simulink model "H2_LQG_quarter_Car"  (R2025b)
settings: Solver=VariableStepAuto  StartTime=0.0  StopTime=30  RelTol=1e-3
values from neighbouring files (symbols this model uses):
  omega_n1 = 80    [A_quarter_car_parameters.m]    (also in A_uncertain_Plant.m = parameters.omega_n1; Incert_plant.m; LQG.m; LQG_pt2.m)
  tau_1 = 0.005    [A_quarter_car_parameters.m]    (also in LQG.m; LQG_pt2.m; LQG_pt2.mat; Lin_model.m)
  tau_2 = 0.010    (= 0.01)    [A_quarter_car_parameters.m]    (also in LQG.m; LQG_pt2.m; LQG_pt2.mat; Lin_model.m)
  tau_a = 0.025    [A_quarter_car_parameters.m]    (also in A_uncertain_Plant.m = parameters.tau_a; Incert_plant.m; LQG.m; LQG_pt2.m)
  x0_delta_s = 0    [A_quarter_car_parameters.m]    (also in quarter_car_parameters.m)
  x0_delta_t = 0    [A_quarter_car_parameters.m]    (also in quarter_car_parameters.m)
  x0_zs_dot = 0    [A_quarter_car_parameters.m]    (also in quarter_car_parameters.m)
  x0_zu_dot = 0    [A_quarter_car_parameters.m]    (also in quarter_car_parameters.m)
  zeta_1 = 0.7    [A_quarter_car_parameters.m]    (also in A_uncertain_Plant.m = parameters.zeta_1; Incert_plant.m; LQG.m; LQG_pt2.m)
libraries: simulink x4, cstblocks x3
settings Model: Creator=ettor  LastModifiedBy=ettor

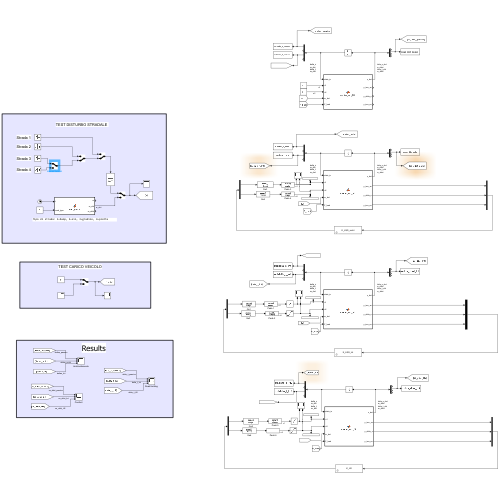
[thumbnail: Simulink's stored preview of the top-level diagram]
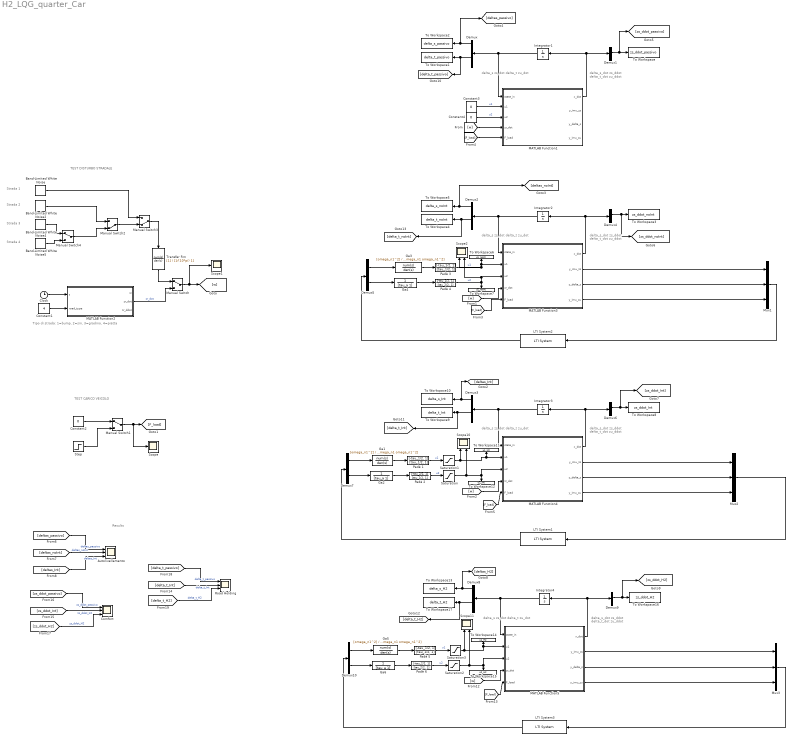
== system H2_LQG_quarter_Car ==
  note: Results
  note: Tipo di strada: 1=bump, 2=sin, 3=gradino, 4=piatta
  note: TEST CARICO VEICOLO
  note: delta_s
      | zs_dot
      | delta_t
      | zu_dot
  note: delta_s_dot
      | zs_ddot
      | delta_t_dot
      | zu_ddot
  note: delta_s_dot
      | zs_ddot
      | delta_t_dot
      | zu_ddot
  note: TEST DISTURBO STRADALE
  note: delta_s_dot
      | zs_ddot
      | delta_t_dot
      | zu_ddot
  note: delta_s
      | zs_dot
      | delta_t
      | zu_dot
  note: delta_s
      | zs_dot
      | delta_t
      | zu_dot
  note: delta_s_dot
      | zs_ddot
      | delta_t_dot
      | zu_ddot
  note: delta_s
      | zs_dot
      | delta_t
      | zu_dot
  note: Strada 2
  note: Strada 3
  note: Strada 4
  note: Strada 1
  Autolivellamento : Scope  NumInputPorts=3
      settings: ActiveDisplayYMinimum=-0.18076927505597792  ActiveDisplayYMaximum=0.021014396276541246  YLabel=[m]  DataLoggingVariableName=ScopeData2
  Band-Limited White Noise : simulink/Sources/Band-Limited White Noise  Cov=[5e-3*0.01]  Ts=0.01  seed=[23341]
  Band-Limited White Noise2 : simulink/Sources/Band-Limited White Noise  Cov=[6e-2*0.01]  Ts=0.01  seed=[23341]
  Band-Limited White Noise4 : simulink/Sources/Band-Limited White Noise  Cov=[0.15*0.01]  Ts=0.01  seed=[23341]
  Band-Limited White Noise5 : simulink/Sources/Band-Limited White Noise  Cov=[0.30*0.01]  Ts=0.01  seed=[23341]
  Clock : Clock
  "Comfort " : Scope  NumInputPorts=3
      settings: ActiveDisplayYMinimum=-3.7790657356038841  ActiveDisplayYMaximum=3.5650054973377014  YLabel=[m/s^2]  DataLoggingVariableName=ScopeData8
  Constant1 : Constant  Value=4
  Constant2 : Constant  Value=0
  Constant3 : Constant  Value=0
  Constant4 : Constant  Value=0
  Demux{,1..4,6,8..9} (8 alike) : Demux
  Demux10 : Demux  Outputs=2
  Demux5 : Demux  Outputs=2
  Demux7 : Demux  Outputs=2
  Ga1 : TransferFcn  Numerator=[omega_n1^2]  Denominator=[1 2*zeta_1*omega_n1 omega_n1^2]
  Ga2 : TransferFcn  Denominator=[tau_a 1]
  Ga3 : TransferFcn  Numerator=[omega_n1^2]  Denominator=[1 2*zeta_1*omega_n1 omega_n1^2]
  Ga4 : TransferFcn  Denominator=[tau_a 1]
  Ga5 : TransferFcn  Numerator=[omega_n1^2]  Denominator=[1 2*zeta_1*omega_n1 omega_n1^2]
  Ga6 : TransferFcn  Denominator=[tau_a 1]
  Integrator{1..4} (4 alike) : Integrator  InitialCondition=[x0_delta_s; x0_zs_dot; x0_delta_t; x0_zu_dot]
  LTI System1 : cstblocks/LTI System  sys=K_LQG_Int  IC=[]  PadeOrder=0
  LTI System2 : cstblocks/LTI System  sys=K_LQG_noInt  IC=[]  PadeOrder=0
  LTI System3 : cstblocks/LTI System  sys=K_H2  IC=[]  PadeOrder=0
  MATLAB Function1 : MATLAB Function  TreatAsAtomicUnit=on
  MATLAB Function2 : MATLAB Function  TreatAsAtomicUnit=on
  MATLAB Function3 : MATLAB Function  TreatAsAtomicUnit=on
  MATLAB Function4 : MATLAB Function  TreatAsAtomicUnit=on
  MATLAB Function5 : MATLAB Function  TreatAsAtomicUnit=on
  Manual Switch : ManualSwitch
  Manual Switch1 : ManualSwitch
  Manual Switch2 : ManualSwitch  CurrentSetting=0
  Manual Switch3 : ManualSwitch  CurrentSetting=0
  Manual Switch4 : ManualSwitch
  Mux1 : Mux  Inputs=3
  Mux2 : Mux  Inputs=3
  Mux3 : Mux  Inputs=3
  Padè 1 : TransferFcn  Numerator=[-tau_1/2, 1]  Denominator=[tau_1/2, 1]
  Padè 2 : TransferFcn  Numerator=[-tau_2/2, 1]  Denominator=[tau_2/2, 1]
  Padè 3 : TransferFcn  Numerator=[-tau_1/2, 1]  Denominator=[tau_1/2, 1]
  Padè 4 : TransferFcn  Numerator=[-tau_2/2, 1]  Denominator=[tau_2/2, 1]
  Padè 5 : TransferFcn  Numerator=[-tau_1/2, 1]  Denominator=[tau_1/2, 1]
  Padè 6 : TransferFcn  Numerator=[-tau_2/2, 1]  Denominator=[tau_2/2, 1]
  "Road Holding " : Scope  NumInputPorts=3
      settings: ActiveDisplayYMinimum=-0.017632393466422407  ActiveDisplayYMaximum=0.022207758401506367  YLabel=[m]  DataLoggingVariableName=ScopeData11
  Saturation : Saturate  UpperLimit=+3000  LowerLimit=-3000
  Saturation1 : Saturate  UpperLimit=+3000  LowerLimit=-3000
  Saturation2 : Saturate  UpperLimit=+10000  LowerLimit=-10000
  Saturation3 : Saturate  UpperLimit=+5000  LowerLimit=-5000
  Scope : Scope
      settings: ActiveDisplayYMinimum=-1  ActiveDisplayYMaximum=1
  Scope1 : Scope
      settings: ActiveDisplayYMinimum=-1  ActiveDisplayYMaximum=1
  Scope10 : Scope  NumInputPorts=2
      settings: ActiveDisplayYMinimum=-1  ActiveDisplayYMaximum=1  DataLoggingVariableName=ScopeData9
  Scope11 : Scope  NumInputPorts=2
      settings: ActiveDisplayYMinimum=-103.06262892158483  ActiveDisplayYMaximum=567.88180424316226  DataLoggingVariableName=ScopeData10
  Scope2 : Scope  NumInputPorts=2
      settings: ActiveDisplayYMinimum=-1  ActiveDisplayYMaximum=1  DataLoggingVariableName=ScopeData3
  Step : Step  After=1000  SampleTime=0
  To Workspace : ToWorkspace  VariableName=zs_ddot_passivo  SaveFormat=Timeseries  SampleTime=-1
  To Workspace1 : ToWorkspace  VariableName=delta_t_passivo  SaveFormat=Timeseries  SampleTime=-1
  To Workspace10 : ToWorkspace  VariableName=delta_s_Int  SaveFormat=Timeseries  SampleTime=-1
  To Workspace11 : ToWorkspace  VariableName=u1_Int  SaveFormat=Timeseries  SampleTime=-1
  To Workspace12 : ToWorkspace  VariableName=u2_Int  SaveFormat=Timeseries  SampleTime=-1
  To Workspace13 : ToWorkspace  VariableName=delta_s_H2  SaveFormat=Timeseries  SampleTime=-1
  To Workspace14 : ToWorkspace  VariableName=u1_H2  SaveFormat=Timeseries  SampleTime=-1
  To Workspace15 : ToWorkspace  VariableName=u2_H2  SaveFormat=Timeseries  SampleTime=-1
  To Workspace16 : ToWorkspace  VariableName=zs_ddot_H2  SaveFormat=Timeseries  SampleTime=-1
  To Workspace17 : ToWorkspace  VariableName=delta_t_H2  SaveFormat=Timeseries  SampleTime=-1
  To Workspace2 : ToWorkspace  VariableName=delta_s_passivo  SaveFormat=Timeseries  SampleTime=-1
  To Workspace3 : ToWorkspace  VariableName=zs_ddot_noInt  SaveFormat=Timeseries  SampleTime=-1
  To Workspace4 : ToWorkspace  VariableName=delta_t_noInt  SaveFormat=Timeseries  SampleTime=-1
  To Workspace5 : ToWorkspace  VariableName=delta_s_noInt  SaveFormat=Timeseries  SampleTime=-1
  To Workspace6 : ToWorkspace  VariableName=u1_noInt  SaveFormat=Timeseries  SampleTime=-1
  To Workspace7 : ToWorkspace  VariableName=u2_noInt  SaveFormat=Timeseries  SampleTime=-1
  To Workspace8 : ToWorkspace  VariableName=zs_ddot_Int  SaveFormat=Timeseries  SampleTime=-1
  To Workspace9 : ToWorkspace  VariableName=delta_t_Int  SaveFormat=Timeseries  SampleTime=-1
  Transfer Fcn : TransferFcn  Denominator=[1/(10*pi) 1]
  wires:
  Manual Switch1/1 -> Scope/1, [F_load]
  Ga3/1 -> Padè 3/1
  Step/1 -> Manual Switch1/2
  Demux5/2 -> Ga4/1
  Saturation1/1 -> To Workspace11/1, MATLAB Function4/2(u1), Scope10/1
  Padè 1/1 -> Saturation1/1  "u1"
  Demux3/1 -> [deltas_Int], To Workspace10/1
  Demux3/3 -> [delta_t_Int], To Workspace9/1
  Demux2/1 -> [deltas_noInt], To Workspace5/1
  Demux7/2 -> Ga2/1
  Demux4/2 -> [zs_ddot_noInt], To Workspace3/1
  Constant2/1 -> Manual Switch1/1
  MATLAB Function2/2(zr_dot) -> Manual Switch/2  "zr_dot"
  [F_load] -> MATLAB Function4/5(F_load)
  Mux1/1 -> LTI System2/1
  MATLAB Function1/1(x_dot) -> Integrator1/1, Demux1/1
  Demux/1 -> [deltas_passivo], To Workspace2/1
  Integrator2/1 -> MATLAB Function3/1(state_in), Demux2/1
  Ga1/1 -> Padè 1/1
  Saturation/1 -> To Workspace12/1, MATLAB Function4/3(u2), Scope10/2
  [w] -> MATLAB Function3/4(zr_dot)
  Demux5/1 -> Ga3/1
  Demux/3 -> [delta_t_passivo], To Workspace1/1
  Integrator1/1 -> MATLAB Function1/1(state_in), Demux/1
  Demux6/2 -> [zs_ddot_Int], To Workspace8/1
  Constant1/1 -> MATLAB Function2/2(road_type)
  Constant4/1 -> MATLAB Function1/3(u2)  "u2"
  MATLAB Function3/1(x_dot) -> Demux4/1, Integrator2/1
  LTI System2/1 -> Demux5/1
  Padè 4/1 -> Scope2/2, MATLAB Function3/3(u2), To Workspace7/1  "u2"
  Padè 2/1 -> Saturation/1  "u2"
  [w] -> MATLAB Function4/4(zr_dot)
  Ga2/1 -> Padè 2/1
  Constant3/1 -> MATLAB Function1/2(u1)  "u1"
  [F_load] -> MATLAB Function3/5(F_load)
  [F_load] -> MATLAB Function1/5(F_load)
  Padè 3/1 -> Scope2/1, To Workspace6/1, MATLAB Function3/2(u1)  "u1"
  [w] -> MATLAB Function1/4(zr_dot)
  Mux2/1 -> LTI System1/1
  Demux2/3 -> [delta_t_noInt], To Workspace4/1
  Integrator3/1 -> MATLAB Function4/1(state_in), Demux3/1
  Demux7/1 -> Ga1/1
  Clock/1 -> MATLAB Function2/1(t)
  Demux1/2 -> [zs_ddot_passivo], To Workspace/1
  MATLAB Function4/1(x_dot) -> Demux6/1, Integrator3/1
  Ga4/1 -> Padè 4/1
  LTI System1/1 -> Demux7/1
  Manual Switch/1 -> Scope1/1, [w]
  [deltas_passivo] -> Autolivellamento/1  "deltas_passivo"
  [deltas_noInt] -> Autolivellamento/2  "deltas_noInt"
  [deltas_Int] -> Autolivellamento/3  "deltas_Int"
  Band-Limited White Noise/1 -> Manual Switch3/1
  Band-Limited White Noise2/1 -> Manual Switch2/1
  Manual Switch2/1 -> Manual Switch3/2
  Manual Switch3/1 -> Transfer Fcn/1
  Ga5/1 -> Padè 5/1
  [F_load] -> MATLAB Function5/5(F_load)
  Demux10/2 -> Ga6/1
  Demux8/3 -> [delta_t_H2], To Workspace17/1
  Saturation2/1 -> MATLAB Function5/3(u2), To Workspace15/1, Scope11/2
  Demux8/1 -> [deltas_H2], To Workspace13/1
  Padè 5/1 -> Saturation3/1  "u1"
  Saturation3/1 -> To Workspace14/1, MATLAB Function5/2(u1), Scope11/1
  Demux10/1 -> Ga5/1
  Integrator4/1 -> MATLAB Function5/1(state_in), Demux8/1
  Mux3/1 -> LTI System3/1
  Ga6/1 -> Padè 6/1
  Padè 6/1 -> Saturation2/1  "u2"
  Demux9/2 -> [zs_ddot_H2], To Workspace16/1
  LTI System3/1 -> Demux10/1
  MATLAB Function5/1(x_dot) -> Demux9/1, Integrator4/1
  [w] -> MATLAB Function5/4(zr_dot)
  [zs_ddot_passivo] -> "Comfort "/1  "zs_ddot_passivo"
  [zs_ddot_Int] -> "Comfort "/2  "zs_ddot_Int"
  [zs_ddot_H2] -> "Comfort "/3  "zs_ddot_H2"
  [delta_t_passivo] -> "Road Holding "/1  "delta_t_passivo"
  [delta_t_Int] -> "Road Holding "/2  "delta_t_Int"
  [delta_t_H2] -> "Road Holding "/3  "delta_t_H2"
  Transfer Fcn/1 -> Manual Switch/1
  Manual Switch4/1 -> Manual Switch2/2
  Band-Limited White Noise4/1 -> Manual Switch4/1
  Band-Limited White Noise5/1 -> Manual Switch4/2
  MATLAB Function4/2(y_imu_zs) -> Mux2/1
  MATLAB Function4/3(y_delta_s) -> Mux2/2
  MATLAB Function4/4(y_imu_zu) -> Mux2/3
  MATLAB Function3/2(y_imu_zs) -> Mux1/1
  MATLAB Function3/3(y_delta_s) -> Mux1/2
  MATLAB Function3/4(y_imu_zu) -> Mux1/3
  MATLAB Function5/2(y_imu_zs) -> Mux3/1
  MATLAB Function5/3(y_delta_s) -> Mux3/2
  MATLAB Function5/4(y_imu_zu) -> Mux3/3

== matlab function H2_LQG_quarter_Car/MATLAB Function1 ==
  data: state_in input; x_dot output; u1 input; u2 input; zr_dot input; F_load input; parameters parameter; y_imu_zs output; y_delta_s output; y_imu_zu output
function [x_dot,y_imu_zs, y_delta_s , y_imu_zu ] = quarter_car_NL(state_in, u1, u2, zr_dot, F_load ,parameters)

    delta_s = state_in(1);
    zs_dot = state_in(2);
    delta_t = state_in(3);
    zu_dot = state_in(4);
    
    m_s = parameters.m_s;
    m_u = parameters.m_u;
    ks0 = parameters.ks0;
    alpha = parameters.alpha;
    bs = parameters.bs;
    kt = parameters.kt;
    bt = parameters.bt;
    
    delta_s_dot = zs_dot - zu_dot;
    delta_t_dot = zu_dot - zr_dot;
    
    Fs = ks0 * delta_s + alpha * delta_s^3 + bs * delta_s_dot;
    Ft = kt * delta_t + bt * delta_t_dot;
    
    
    zs_ddot = (-Fs + u1-F_load) / m_s;
    zu_ddot = (Fs - Ft - u1 + u2) / m_u;
    
    x_dot = [delta_s_dot; zs_ddot; delta_t_dot; zu_ddot];
    
    y_imu_zs = zs_ddot; 
    y_imu_zu = zu_ddot;
    y_delta_s = delta_s; % Sensore di altezza (Ride Height) 

end

== matlab function H2_LQG_quarter_Car/MATLAB Function4 ==
  data: state_in input; x_dot output; u1 input; u2 input; zr_dot input; F_load input; parameters parameter; y_imu_zs output; y_delta_s output; y_imu_zu output
function [x_dot,y_imu_zs, y_delta_s , y_imu_zu ] = quarter_car_NL(state_in, u1, u2, zr_dot, F_load ,parameters)

    delta_s = state_in(1);
    zs_dot = state_in(2);
    delta_t = state_in(3);
    zu_dot = state_in(4);
    
    m_s = parameters.m_s;
    m_u = parameters.m_u;
    ks0 = parameters.ks0;
    alpha = parameters.alpha;
    bs = parameters.bs;
    kt = parameters.kt;
    bt = parameters.bt;
    
    delta_s_dot = zs_dot - zu_dot;
    delta_t_dot = zu_dot - zr_dot;
    
    Fs = ks0 * delta_s + alpha * delta_s^3 + bs * delta_s_dot;
    Ft = kt * delta_t + bt * delta_t_dot;
    
    
    zs_ddot = (-Fs + u1-F_load) / m_s;
    zu_ddot = (Fs - Ft - u1 + u2) / m_u;
    
    x_dot = [delta_s_dot; zs_ddot; delta_t_dot; zu_ddot];
    
    y_imu_zs = zs_ddot; 
    y_imu_zu = zu_ddot;
    y_delta_s = delta_s; % Sensore di altezza (Ride Height) 

end

== matlab function H2_LQG_quarter_Car/MATLAB Function2 ==
  data: t input; zr output; zr_dot output; zr_ddot output; params parameter; road_type input
function [zr, zr_dot, zr_ddot] = road_profile(t, params, road_type)
%   road_type = 1 bump | 2 sinusoide | 3 gradino | 4 piatta

    switch road_type
        case 1  % ---- BUMP ----

            A = params.A;   % altezza [m]
            L = params.L;   % lunghezza [m]
            v = params.v;   % velocità veicolo [m/s]
            t0 = params.t0; % istante di inizio ostacolo [s]
            T = L / v;      % durata temporale bump
            
            % Il dosso inizia a t0 e finisce a t0 + T
            if t >= t0 && t <= (t0 + T)
                t_rel = t - t0; % Tempo relativo (parte da 0 quando inizia il dosso)
                phi   = 2*pi*v*t_rel / L;
                zr    = (A/2) * (1 - cos(phi));
                zr_dot   = (A*pi*v/L) * sin(phi);
                zr_ddot  = (A*2*pi^2*v^2/L^2) * cos(phi);
            else
                zr = 0;  zr_dot = 0;  zr_ddot = 0;
            end
            
        case 2  % ---- SINUSOIDE ----
            A = params.A;   % ampiezza [m]
            f = params.f;   % frequenza [Hz]
            t0 = params.t0; % istante di inizio ostacolo [s]
            
            % La strada vibra solo dopo t0
            if t >= t0
                t_rel = t - t0; % Tempo relativo
                w = 2*pi*f;
                zr   =  A * sin(w*t_rel);
                zr_dot  =  A * w * cos(w*t_rel);
                zr_ddot = -A * w^2 * sin(w*t_rel);
            else
                zr = 0;  zr_dot = 0;  zr_ddot = 0;
            end
            
        case 3  % ---- GRADINO SMUSSATO ----
            A  = params.A;    % altezza [m]
            t0 = params.t0;   % istante del gradino [s]
            tau = params.tau/1000; % tempo di salita [s]
            
            arg  = (t - t0) / tau;
            zr   = (A/2) * (1 + tanh(arg));
            zr_dot  = (A/(2*tau)) * (sech(arg))^2;
            zr_ddot = -(A/tau^2) * (sech(arg))^2 * tanh(arg);
            
        case 4  % ---- STRADA PIATTA ----
            zr = 0;  zr_dot = 0;  zr_ddot = 0;
            
        otherwise 
            zr = 0;  zr_dot = 0;  zr_ddot = 0;
    end
end

== matlab function H2_LQG_quarter_Car/MATLAB Function3 ==
  data: state_in input; x_dot output; u1 input; u2 input; zr_dot input; F_load input; parameters parameter; y_imu_zs output; y_delta_s output; y_imu_zu output
function [x_dot,y_imu_zs, y_delta_s , y_imu_zu ] = quarter_car_NL(state_in, u1, u2, zr_dot, F_load ,parameters)

    delta_s = state_in(1);
    zs_dot = state_in(2);
    delta_t = state_in(3);
    zu_dot = state_in(4);
    
    m_s = parameters.m_s;
    m_u = parameters.m_u;
    ks0 = parameters.ks0;
    alpha = parameters.alpha;
    bs = parameters.bs;
    kt = parameters.kt;
    bt = parameters.bt;
    
    delta_s_dot = zs_dot - zu_dot;
    delta_t_dot = zu_dot - zr_dot;
    
    Fs = ks0 * delta_s + alpha * delta_s^3 + bs * delta_s_dot;
    Ft = kt * delta_t + bt * delta_t_dot;
    
    
    zs_ddot = (-Fs + u1-F_load) / m_s;
    zu_ddot = (Fs - Ft - u1 + u2) / m_u;
    
    x_dot = [delta_s_dot; zs_ddot; delta_t_dot; zu_ddot];
    
    y_imu_zs = zs_ddot; 
    y_imu_zu = zu_ddot;
    y_delta_s = delta_s; % Sensore di altezza (Ride Height) 

end

== matlab function H2_LQG_quarter_Car/MATLAB Function5 ==
  data: state_in input; x_dot output; u1 input; u2 input; zr_dot input; F_load input; parameters parameter; y_imu_zs output; y_delta_s output; y_imu_zu output
function [x_dot,y_imu_zs, y_delta_s , y_imu_zu ] = quarter_car_NL(state_in, u1, u2, zr_dot, F_load ,parameters)

    delta_s = state_in(1);
    zs_dot = state_in(2);
    delta_t = state_in(3);
    zu_dot = state_in(4);
    
    m_s = parameters.m_s;
    m_u = parameters.m_u;
    ks0 = parameters.ks0;
    alpha = parameters.alpha;
    bs = parameters.bs;
    kt = parameters.kt;
    bt = parameters.bt;
    
    delta_s_dot = zs_dot - zu_dot;
    delta_t_dot = zu_dot - zr_dot;
    
    Fs = ks0 * delta_s + alpha * delta_s^3 + bs * delta_s_dot;
    Ft = kt * delta_t + bt * delta_t_dot;
    
    
    zs_ddot = (-Fs + u1-F_load) / m_s;
    zu_ddot = (Fs - Ft - u1 + u2) / m_u;
    
    x_dot = [delta_s_dot; zs_ddot; delta_t_dot; zu_ddot];
    
    y_imu_zs = zs_ddot; 
    y_imu_zu = zu_ddot;
    y_delta_s = delta_s; % Sensore di altezza (Ride Height) 

end
